simulink model "Climate_Control"  (R2020a)
settings: Solver=FixedStepDiscrete  StartTime=0.0  StopTime=35  FixedStep=1  RelTol=1e-3
libraries: simulink x1
settings Model: Creator=ashok  LastModifiedBy=ashok
settings DataIOCC: ExternalInput=[t, T]

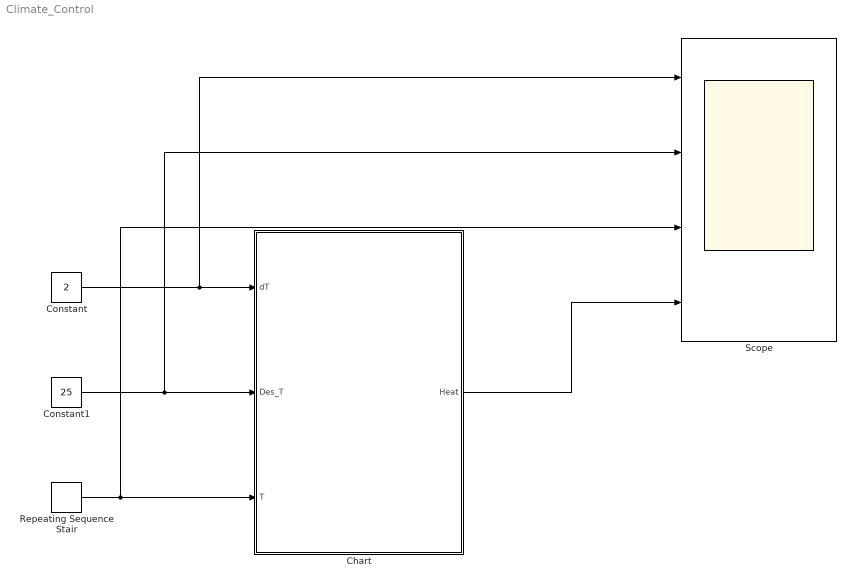
== system Climate_Control ==
  Chart : Stateflow chart  TreatAsAtomicUnit=on
  Constant : Constant  Value=2
  Constant1 : Constant  Value=25
  Repeating Sequence Stair : simulink/Sources/Repeating Sequence Stair  OutValues=T  tsamp=-1  OutMin=[]  OutMax=[]  OutDataTypeStr=double  OutputDataTypeScalingMode=double  OutDataType=fixdt(0,8)  ConRadixGroup=Best Precision: Vector-wise  OutScaling=2^-12
  Scope : Scope  NumInputPorts=4
  wires:
  Constant/1 -> Scope/1, Chart/1(dT)
  Constant1/1 -> Scope/2, Chart/2(Des_T)
  Repeating Sequence Stair/1 -> Scope/3, Chart/3(T)
  Chart/1(Heat) -> Scope/4

== stateflow chart Climate_Control/Chart ==
  state OFF
    en:
    Heat = 0;
  state WARM
    en:
    Heat = 1;
  state COOL
    en:
    Heat = -1;
  (default) -> (junction 8)
  (junction 8) -> WARM [order 2] : [T <= (Des_T - dT)]
  (junction 8) -> COOL [order 1] : [T >= (Des_T + dT)]
  (junction 8) -> OFF [order 3]
  OFF -> COOL [order 2] : [T >= (Des_T + dT) ]
  OFF -> WARM [order 1] : [T <= (Des_T - dT) ]
  WARM -> OFF : [T >= (Des_T - dT) ]
  COOL -> OFF : [T <= (Des_T + dT) ]
  data: dT input; Des_T input; T input; Heat output
